simulink model "ADMIRE"  (R2021b)
settings: Solver=ode4  StartTime=0.0  StopTime=100  FixedStep=1e-2  RelTol=1e-3
undefined symbols (not defined in the file or in its folder): admireDB, Earth, WGS84
libraries: simulink_extras x112, simulink x27, aerolibutil x4, dspsigops x4, aerolibfltsims x3, sharedtransform x2, aerolibtransform2 x2, aerolibatmos2 x1, matrix_library x1, sharedutil x1, aerolibanimutils x1, vrlib x1
(part 6 of 15)

== system ADMIRE/Aircraft/Aerodynamics/PitchMomentCoefficient/MachRegion3/Cpmalfa ==
  in_bus : Inport
  Bus Selector : BusSelector  OutputSignals=AeroIn_Bus.angleOfAttack_deg,AeroIn_Bus.mach_nd,AeroIn_Bus.qacorr
  CPMEA_QA_M : Lookup_n-D  BreakpointsForDimension1=admireDB.aerodata_sym.CPMEA.breakpoints.M  BreakpointsForDimension2=admireDB.aerodata_sym.CPMEA.breakpoints.QA  BreakpointsForDimension3=[5, 7]  Table=admireDB.aerodata_sym.CPMEA.newTable  ExtrapMethod=Clip  InternalRulePriority=Speed  RndMeth=Simplest  InputSameDT=on
      settings: InputPortMap=u0,u1
  CPMMDEA_ALFA_DE_M : Lookup_n-D  NumberOfTableDimensions=3  BreakpointsForDimension1=admireDB.aerodata_sym.CPMMDEA.breakpoints.ALFA  BreakpointsForDimension2=admireDB.aerodata_sym.CPMMDEA.breakpoints.DE  BreakpointsForDimension3=admireDB.aerodata_sym.CPMMDEA.breakpoints.M  Table=admireDB.aerodata_sym.CPMMDEA.newTable  ExtrapMethod=Clip  InternalRulePriority=Speed  RndMeth=Simplest  InputSameDT=on
      settings: InputPortMap=u0,u1,u2
  Degrees to Radians : simulink_extras/Transformations/Degrees to Radians
  Product : Product
  Sum1 : Sum  Inputs=|++
  dE_cnst : Constant  Value=0.0
  Cpmalfa : Outport
  wires:
  Product/1 -> Sum1/2
  CPMMDEA_ALFA_DE_M/1 -> Sum1/1
  Sum1/1 -> Cpmalfa/1
  in_bus/1 -> Bus Selector/1  "in_bus"
  Bus Selector/1 -> CPMMDEA_ALFA_DE_M/1, Degrees to Radians/1  "<angleOfAttack_deg>"
  dE_cnst/1 -> CPMMDEA_ALFA_DE_M/2
  Bus Selector/3 -> CPMEA_QA_M/2  "<qacorr>"
  Bus Selector/2 -> CPMMDEA_ALFA_DE_M/3, CPMEA_QA_M/1  "<mach_nd>"
  CPMEA_QA_M/1 -> Product/2
  Degrees to Radians/1 -> Product/1

== system ADMIRE/Aircraft/Aerodynamics/PitchMomentCoefficient/MachRegion3/Cpmalfad ==
  in_bus : Inport
  Abs : Abs
  Bus Selector : BusSelector  OutputSignals=AeroIn_Bus.mach_nd,AeroIn_Bus.angleOfAttack_deg,AeroIn_Bus.alfad
  CPMADAM_ALFA_M : Lookup_n-D  BreakpointsForDimension1=admireDB.aerodata_sym.CPMADAM.breakpoints.M  BreakpointsForDimension2=admireDB.aerodata_sym.CPMADAM.breakpoints.ALFA  BreakpointsForDimension3=[5, 7]  Table=admireDB.aerodata_sym.CPMADAM.newTable  ExtrapMethod=Clip  InternalRulePriority=Speed  RndMeth=Simplest  InputSameDT=on
      settings: InputPortMap=u0,u1
  Product : Product
  Cpmalfad : Outport
  wires:
  in_bus/1 -> Bus Selector/1  "in_bus"
  Bus Selector/2 -> Abs/1  "<angleOfAttack_deg>"
  Bus Selector/1 -> CPMADAM_ALFA_M/1  "<mach_nd>"
  Abs/1 -> CPMADAM_ALFA_M/2
  CPMADAM_ALFA_M/1 -> Product/1
  Bus Selector/3 -> Product/2  "<alfad>"
  Product/1 -> Cpmalfad/1

== system ADMIRE/Aircraft/Aerodynamics/PitchMomentCoefficient/MachRegion3/Cpmbasic ==
  in_bus : Inport
  Bus Selector : BusSelector  OutputSignals=AeroIn_Bus.mach_nd,AeroIn_Bus.qacorr
  CPMEZERO_QA_M : Lookup_n-D  BreakpointsForDimension1=admireDB.aerodata_sym.CPMEZERO.breakpoints.M  BreakpointsForDimension2=admireDB.aerodata_sym.CPMEZERO.breakpoints.QA  BreakpointsForDimension3=[5, 7]  Table=admireDB.aerodata_sym.CPMEZERO.newTable  ExtrapMethod=Clip  InternalRulePriority=Speed  RndMeth=Simplest  InputSameDT=on
      settings: InputPortMap=u0,u1
  CPMZERO_M : Lookup_n-D  NumberOfTableDimensions=1  BreakpointsForDimension1=admireDB.aerodata_sym.CPMZERO.breakpoints.M  BreakpointsForDimension3=[5, 7]  Table=admireDB.aerodata_sym.CPMZERO.newTable  ExtrapMethod=Clip  InternalRulePriority=Speed  RndMeth=Simplest  InputSameDT=on
  Sum1 : Sum  Inputs=|++
  Cpmbasic : Outport
  wires:
  in_bus/1 -> Bus Selector/1  "in_bus"
  Sum1/1 -> Cpmbasic/1
  Bus Selector/1 -> CPMZERO_M/1, CPMEZERO_QA_M/1  "<mach_nd>"
  Bus Selector/2 -> CPMEZERO_QA_M/2  "<qacorr>"
  CPMZERO_M/1 -> Sum1/1
  CPMEZERO_QA_M/1 -> Sum1/2

== system ADMIRE/Aircraft/Aerodynamics/PitchMomentCoefficient/MachRegion3/Cpmbeta ==
  Constant : Constant  Value=0
  Cpmbeta : Outport
  wires:
  Constant/1 -> Cpmbeta/1

== system ADMIRE/Aircraft/Aerodynamics/PitchMomentCoefficient/MachRegion3/Cpmcai ==
  in_bus : Inport
  Bus Selector : BusSelector  OutputSignals=AeroIn_Bus.angleOfAttack_deg,AeroIn_Bus.cai,AeroIn_Bus.dN
  CPMCAIDN_ALFA_CAI_DN : Lookup_n-D  NumberOfTableDimensions=3  BreakpointsForDimension1=admireDB.aerodata_sym.CPMCAIDN.breakpoints.ALFA  BreakpointsForDimension2=admireDB.aerodata_sym.CPMCAIDN.breakpoints.CAI  BreakpointsForDimension3=admireDB.aerodata_sym.CPMCAIDN.breakpoints.DN  Table=admireDB.aerodata_sym.CPMCAIDN.newTable  ExtrapMethod=Clip  InternalRulePriority=Speed  RndMeth=Simplest  InputSameDT=on
      settings: InputPortMap=u0,u1,u2
  CPMCAI_CAI_ALFA : Lookup_n-D  BreakpointsForDimension1=admireDB.aerodata_sym.CPMCAI.breakpoints.ALFA  BreakpointsForDimension2=admireDB.aerodata_sym.CPMCAI.breakpoints.CAI  BreakpointsForDimension3=[5, 7]  Table=admireDB.aerodata_sym.CPMCAI.newTable  ExtrapMethod=Clip  InternalRulePriority=Speed  RndMeth=Simplest  InputSameDT=on
      settings: InputPortMap=u0,u1
  Sum : Sum  Inputs=|++
  Cpmcai : Outport
  wires:
  Bus Selector/3 -> CPMCAIDN_ALFA_CAI_DN/3  "<dN>"
  CPMCAI_CAI_ALFA/1 -> Sum/1
  Bus Selector/2 -> CPMCAI_CAI_ALFA/2, CPMCAIDN_ALFA_CAI_DN/2  "<cai>"
  Bus Selector/1 -> CPMCAI_CAI_ALFA/1, CPMCAIDN_ALFA_CAI_DN/1  "<angleOfAttack_deg>"
  in_bus/1 -> Bus Selector/1  "in_bus"
  Sum/1 -> Cpmcai/1
  CPMCAIDN_ALFA_CAI_DN/1 -> Sum/2

== system ADMIRE/Aircraft/Aerodynamics/PitchMomentCoefficient/MachRegion3/Cpmda ==
  Constant : Constant  Value=0
  Cpmda : Outport
  wires:
  Constant/1 -> Cpmda/1

== system ADMIRE/Aircraft/Aerodynamics/PitchMomentCoefficient/MachRegion3/Cpmdedn ==
  Constant : Constant  Value=0
  Cpmdedn : Outport
  wires:
  Constant/1 -> Cpmdedn/1

== system ADMIRE/Aircraft/Aerodynamics/PitchMomentCoefficient/MachRegion3/Cpmdei ==
  in_bus : Inport
  Bus Selector : BusSelector  OutputSignals=AeroIn_Bus.dEI,AeroIn_Bus.angleOfAttack_deg,eieff,AeroIn_Bus.mach_nd,AeroIn_Bus.qacorr
  CPMEDEI_QA_M : Lookup_n-D  BreakpointsForDimension1=admireDB.aerodata_sym.CPMEDEI.breakpoints.M  BreakpointsForDimension2=admireDB.aerodata_sym.CPMEDEI.breakpoints.QA  BreakpointsForDimension3=[5, 7]  Table=admireDB.aerodata_sym.CPMEDEI.newTable  ExtrapMethod=Clip  InternalRulePriority=Speed  RndMeth=Simplest  InputSameDT=on
      settings: InputPortMap=u0,u1
  Product : Product
  Subsystem : Subsystem
  Cpmdei : Outport
  wires:
  in_bus/1 -> Bus Selector/1  "in_bus"
  Bus Selector/5 -> CPMEDEI_QA_M/2  "<qacorr>"
  Bus Selector/1 -> Subsystem/1(dEI)  "<dEI>"
  Bus Selector/2 -> Subsystem/2(angleOfAttack_deg)  "<angleOfAttack_deg>"
  Bus Selector/3 -> Subsystem/3(eieff)  "<eieff>"
  Bus Selector/4 -> Subsystem/4(mach_nd), CPMEDEI_QA_M/1  "<mach_nd>"
  CPMEDEI_QA_M/1 -> Product/2
  Subsystem/1(Out1) -> Product/1
  Product/1 -> Cpmdei/1

== system ADMIRE/Aircraft/Aerodynamics/PitchMomentCoefficient/MachRegion3/Cpmdey ==
  in_bus : Inport
  Bus Selector : BusSelector  OutputSignals=AeroIn_Bus.dEY,AeroIn_Bus.angleOfAttack_deg,eoeff,AeroIn_Bus.mach_nd,AeroIn_Bus.qacorr
  CPMEDEY_QA_M : Lookup_n-D  BreakpointsForDimension1=admireDB.aerodata_sym.CPMEDEY.breakpoints.M  BreakpointsForDimension2=admireDB.aerodata_sym.CPMEDEY.breakpoints.QA  BreakpointsForDimension3=[5, 7]  Table=admireDB.aerodata_sym.CPMEDEY.newTable  ExtrapMethod=Clip  InternalRulePriority=Speed  RndMeth=Simplest  InputSameDT=on
      settings: InputPortMap=u0,u1
  Product : Product
  Subsystem : Subsystem
  Cpmdey : Outport
  wires:
  Product/1 -> Cpmdey/1
  Subsystem/1(Out1) -> Product/1
  CPMEDEY_QA_M/1 -> Product/2
  Bus Selector/4 -> Subsystem/4(mach_nd), CPMEDEY_QA_M/1  "<mach_nd>"
  Bus Selector/3 -> Subsystem/3(eoeff)  "<eoeff>"
  Bus Selector/2 -> Subsystem/2(angleOfAttack_deg)  "<angleOfAttack_deg>"
  Bus Selector/1 -> Subsystem/1(dEY)  "<dEY>"
  Bus Selector/5 -> CPMEDEY_QA_M/2  "<qacorr>"
  in_bus/1 -> Bus Selector/1  "in_bus"

== system ADMIRE/Aircraft/Aerodynamics/PitchMomentCoefficient/MachRegion3/Cpmdle ==
  in_bus : Inport
  Bus Selector : BusSelector  OutputSignals=AeroIn_Bus.angleOfAttack_deg,AeroIn_Bus.lef_deg,AeroIn_Bus.qacorr,AeroIn_Bus.mach_nd
  CPMMDLEA_ALFA_DLE_M : Lookup_n-D  NumberOfTableDimensions=3  BreakpointsForDimension1=admireDB.aerodata_sym.CPMMDLEA.breakpoints.ALFA  BreakpointsForDimension2=admireDB.aerodata_sym.CPMMDLEA.breakpoints.DLE  BreakpointsForDimension3=admireDB.aerodata_sym.CPMMDLEA.breakpoints.M  Table=admireDB.aerodata_sym.CPMMDLEA.newTable  ExtrapMethod=Clip  InternalRulePriority=Speed  RndMeth=Simplest  InputSameDT=on
      settings: InputPortMap=u0,u1,u2
  Degrees to Radians : simulink_extras/Transformations/Degrees to Radians
  Product : Product
  Subsystem1 : Subsystem
  Sum : Sum  Inputs=|++
  Cpmdle : Outport
  wires:
  in_bus/1 -> Bus Selector/1  "in_bus"
  Bus Selector/1 -> CPMMDLEA_ALFA_DLE_M/1  "<angleOfAttack_deg>"
  Bus Selector/2 -> CPMMDLEA_ALFA_DLE_M/2, Degrees to Radians/1  "<lef_deg>"
  Degrees to Radians/1 -> Product/2
  Product/1 -> Sum/2
  CPMMDLEA_ALFA_DLE_M/1 -> Sum/1
  Sum/1 -> Cpmdle/1
  Bus Selector/3 -> Subsystem1/1(<qacorr>)  "<qacorr>"
  Bus Selector/4 -> Subsystem1/2(<mach_nd>), CPMMDLEA_ALFA_DLE_M/3  "<mach_nd>"
  Subsystem1/1(Out1) -> Product/1

== system ADMIRE/Aircraft/Aerodynamics/PitchMomentCoefficient/MachRegion3/Cpmdn ==
  in_bus : Inport
  Bus Selector : BusSelector  OutputSignals=AeroIn_Bus.angleOfAttack_deg,AeroIn_Bus.dN,AeroIn_Bus.mach_nd,AeroIn_Bus.qacorr
  CPMEDN_QA_M : Lookup_n-D  BreakpointsForDimension1=admireDB.aerodata_sym.CPMEDN.breakpoints.M  BreakpointsForDimension2=admireDB.aerodata_sym.CPMEDN.breakpoints.QA  BreakpointsForDimension3=[5, 7]  Table=admireDB.aerodata_sym.CPMEDN.newTable  ExtrapMethod=Clip  InternalRulePriority=Speed  RndMeth=Simplest  InputSameDT=on
      settings: InputPortMap=u0,u1
  CPMMDNA_ALFA_DN_M : Lookup_n-D  NumberOfTableDimensions=3  BreakpointsForDimension1=admireDB.aerodata_sym.CPMMDNA.breakpoints.ALFA  BreakpointsForDimension2=admireDB.aerodata_sym.CPMMDNA.breakpoints.DN  BreakpointsForDimension3=admireDB.aerodata_sym.CPMMDNA.breakpoints.M  Table=admireDB.aerodata_sym.CPMMDNA.newTable  ExtrapMethod=Clip  InternalRulePriority=Speed  RndMeth=Simplest  InputSameDT=on
      settings: InputPortMap=u0,u1,u2
  Product : Product
  Cpmdn : Outport
  wires:
  Product/1 -> Cpmdn/1
  in_bus/1 -> Bus Selector/1  "in_bus"
  Bus Selector/1 -> CPMMDNA_ALFA_DN_M/1  "<angleOfAttack_deg>"
  Bus Selector/2 -> CPMMDNA_ALFA_DN_M/2  "<dN>"
  Bus Selector/4 -> CPMEDN_QA_M/2  "<qacorr>"
  Bus Selector/3 -> CPMMDNA_ALFA_DN_M/3, CPMEDN_QA_M/1  "<mach_nd>"
  CPMEDN_QA_M/1 -> Product/2
  CPMMDNA_ALFA_DN_M/1 -> Product/1

== system ADMIRE/Aircraft/Aerodynamics/PitchMomentCoefficient/MachRegion3/Cpmhigh ==
  Constant : Constant  Value=0
  Cpmhigh : Outport
  wires:
  Constant/1 -> Cpmhigh/1

== system ADMIRE/Aircraft/Aerodynamics/PitchMomentCoefficient/MachRegion3/Cpmlg ==
  in_bus : Inport
  Abs : Abs
  Bus Selector : BusSelector  OutputSignals=AeroIn_Bus.angleOfAttack_deg,AeroIn_Bus.angleOfSideslip_deg,AeroIn_Bus.lg_bool
  CPMLST_BETA_ALFA : Lookup_n-D  BreakpointsForDimension1=admireDB.aerodata_sym.CPMLST.breakpoints.ALFA  BreakpointsForDimension2=admireDB.aerodata_sym.CPMLST.breakpoints.BETA  BreakpointsForDimension3=[5, 7]  Table=admireDB.aerodata_sym.CPMLST.newTable  ExtrapMethod=Clip  InternalRulePriority=Speed  RndMeth=Simplest  InputSameDT=on
      settings: InputPortMap=u0,u1
  Product : Product
  Cpmlg : Outport
  wires:
  Product/1 -> Cpmlg/1
  in_bus/1 -> Bus Selector/1  "in_bus"
  Bus Selector/1 -> CPMLST_BETA_ALFA/1  "<angleOfAttack_deg>"
  Bus Selector/2 -> Abs/1  "<angleOfSideslip_deg>"
  CPMLST_BETA_ALFA/1 -> Product/1
  Bus Selector/3 -> Product/2  "<lg_bool>"
  Abs/1 -> CPMLST_BETA_ALFA/2

== system ADMIRE/Aircraft/Aerodynamics/PitchMomentCoefficient/MachRegion3/Cpmnz ==
  in_bus : Inport
  Bus Selector : BusSelector  OutputSignals=AeroIn_Bus.nz_g,AeroIn_Bus.mach_nd,AeroIn_Bus.qacorr
  CPMENZ_QA_M : Lookup_n-D  BreakpointsForDimension1=admireDB.aerodata_sym.CPMENZ.breakpoints.M  BreakpointsForDimension2=admireDB.aerodata_sym.CPMENZ.breakpoints.QA  BreakpointsForDimension3=[5, 7]  Table=admireDB.aerodata_sym.CPMENZ.newTable  ExtrapMethod=Clip  InternalRulePriority=Speed  RndMeth=Simplest  InputSameDT=on
      settings: InputPortMap=u0,u1
  Constant : Constant
  Product : Product
  Sum : Sum  Inputs=-+|
  Cpmnz : Outport
  wires:
  in_bus/1 -> Bus Selector/1  "in_bus"
  Sum/1 -> Product/1
  Product/1 -> Cpmnz/1
  Bus Selector/3 -> CPMENZ_QA_M/2  "<qacorr>"
  Bus Selector/2 -> CPMENZ_QA_M/1  "<mach_nd>"
  Bus Selector/1 -> Sum/2  "<nz_g>"
  Constant/1 -> Sum/1
  CPMENZ_QA_M/1 -> Product/2

== system ADMIRE/Aircraft/Aerodynamics/PitchMomentCoefficient/MachRegion3/Cpmq ==
  in_bus : Inport
  Bus Selector : BusSelector  OutputSignals=AeroIn_Bus.qc,AeroIn_Bus.mach_nd,AeroIn_Bus.qacorr,AeroIn_Bus.angleOfAttack_deg
  CPMEQ_QA_M : Lookup_n-D  BreakpointsForDimension1=admireDB.aerodata_sym.CPMEQ.breakpoints.M  BreakpointsForDimension2=admireDB.aerodata_sym.CPMEQ.breakpoints.QA  BreakpointsForDimension3=[5, 7]  Table=admireDB.aerodata_sym.CPMEQ.newTable  ExtrapMethod=Clip  InternalRulePriority=Speed  RndMeth=Simplest  InputSameDT=on
      settings: InputPortMap=u0,u1
  CPMQAM_ALFA_M : Lookup_n-D  BreakpointsForDimension1=admireDB.aerodata_sym.CPMQAM.breakpoints.M  BreakpointsForDimension2=admireDB.aerodata_sym.CPMQAM.breakpoints.ALFA  BreakpointsForDimension3=[5, 7]  Table=admireDB.aerodata_sym.CPMQAM.newTable  ExtrapMethod=Clip  InternalRulePriority=Speed  RndMeth=Simplest  InputSameDT=on
      settings: InputPortMap=u0,u1
  Product : Product  Inputs=3
  Cpmq : Outport
  wires:
  Bus Selector/1 -> Product/1  "<qc>"
  CPMEQ_QA_M/1 -> Product/2
  CPMQAM_ALFA_M/1 -> Product/3
  Product/1 -> Cpmq/1
  in_bus/1 -> Bus Selector/1  "in_bus"
  Bus Selector/4 -> CPMQAM_ALFA_M/2  "<angleOfAttack_deg>"
  Bus Selector/3 -> CPMEQ_QA_M/2  "<qacorr>"
  Bus Selector/2 -> CPMQAM_ALFA_M/1, CPMEQ_QA_M/1  "<mach_nd>"

== system ADMIRE/Aircraft/Aerodynamics/PitchMomentCoefficient/MachRegion3/Cpmqd ==
  in_bus : Inport
  Bus Selector : BusSelector  OutputSignals=AeroIn_Bus.qd,AeroIn_Bus.mach_nd,AeroIn_Bus.qacorr
  CPMEQD_QA_M : Lookup_n-D  BreakpointsForDimension1=admireDB.aerodata_sym.CPMEQD.breakpoints.M  BreakpointsForDimension2=admireDB.aerodata_sym.CPMEQD.breakpoints.QA  BreakpointsForDimension3=[5, 7]  Table=admireDB.aerodata_sym.CPMEQD.newTable  ExtrapMethod=Clip  InternalRulePriority=Speed  RndMeth=Simplest  InputSameDT=on
      settings: InputPortMap=u0,u1
  Product : Product
  Cpmqd : Outport
  wires:
  CPMEQD_QA_M/1 -> Product/2
  Bus Selector/1 -> Product/1  "<qd>"
  Bus Selector/2 -> CPMEQD_QA_M/1  "<mach_nd>"
  Bus Selector/3 -> CPMEQD_QA_M/2  "<qacorr>"
  Product/1 -> Cpmqd/1
  in_bus/1 -> Bus Selector/1  "in_bus"

== system ADMIRE/Aircraft/Aerodynamics/PitchMomentCoefficient/MachRegion3/eoeff ==
  AeroIn_Bus : Inport
  Abs : Abs
  Bus Selector : BusSelector  OutputSignals=mach_nd,angleOfAttack_deg
  CPMDEYOD_ALFA_M : Lookup_n-D  BreakpointsForDimension1=admireDB.aerodata_sym.CPMDEYOD.breakpoints.M  BreakpointsForDimension2=admireDB.aerodata_sym.CPMDEYOD.breakpoints.ALFA  BreakpointsForDimension3=[5, 7]  Table=admireDB.aerodata_sym.CPMDEYOD.newTable  ExtrapMethod=Clip  InternalRulePriority=Speed  RndMeth=Simplest  InputSameDT=on
      settings: InputPortMap=u0,u1
  Constant : Constant
  Sum : Sum  Inputs=-+|
  eoeff : Outport
  eieff : Outport  Port=2
  wires:
  AeroIn_Bus/1 -> Bus Selector/1
  Bus Selector/1 -> CPMDEYOD_ALFA_M/1  "<mach_nd>"
  Constant/1 -> Sum/2
  CPMDEYOD_ALFA_M/1 -> Sum/1, eoeff/1
  Sum/1 -> eieff/1
  Bus Selector/2 -> Abs/1  "<angleOfAttack_deg>"
  Abs/1 -> CPMDEYOD_ALFA_M/2

== system ADMIRE/Aircraft/Aerodynamics/RollMomentCoefficient/MachRegion1/Crmbasic ==
  in_bus : Inport
  Bus Selector : BusSelector  OutputSignals=AeroIn_Bus.angleOfAttack_deg
  Crmbasic_ : Subsystem
  Crmbasic : Outport
  wires:
  Crmbasic_/1(Crmbasic) -> Crmbasic/1
  Bus Selector/1 -> Crmbasic_/1(angleOfAttack_deg)  "<angleOfAttack_deg>"
  in_bus/1 -> Bus Selector/1  "in_bus"

== system ADMIRE/Aircraft/Aerodynamics/RollMomentCoefficient/MachRegion1/Crmbde ==
  in_bus : Inport
  Bus Selector : BusSelector  OutputSignals=AeroIn_Bus.angleOfAttack_deg,AeroIn_Bus.dN,AeroIn_Bus.dEI,AeroIn_Bus.angleOfSideslip_deg,AeroIn_Bus.dEY,eieff,eoeff
  Crmbde_ : Subsystem
  Crmbde : Outport
  wires:
  Bus Selector/7 -> Crmbde_/7(eoeff)  "<eoeff>"
  Bus Selector/6 -> Crmbde_/6(eieff)  "<eieff>"
  Bus Selector/5 -> Crmbde_/5(dEY)  "<dEY>"
  Bus Selector/4 -> Crmbde_/4(angleOfSideslip_deg)  "<angleOfSideslip_deg>"
  Bus Selector/3 -> Crmbde_/3(dEI)  "<dEI>"
  Bus Selector/2 -> Crmbde_/2(dN)  "<dN>"
  Bus Selector/1 -> Crmbde_/1(angleOfAttack_deg)  "<angleOfAttack_deg>"
  Crmbde_/1(Crmbde) -> Crmbde/1
  in_bus/1 -> Bus Selector/1  "in_bus"

== system ADMIRE/Aircraft/Aerodynamics/RollMomentCoefficient/MachRegion1/Crmbdle ==
  in_bus : Inport
  Bus Selector : BusSelector  OutputSignals=AeroIn_Bus.lef_deg,AeroIn_Bus.angleOfSideslip_deg,AeroIn_Bus.dEI,AeroIn_Bus.angleOfAttack_deg,AeroIn_Bus.dEY,eieff,eoeff
  Crmbdle_ : Subsystem
  Crmbdle : Outport
  wires:
  Bus Selector/7 -> Crmbdle_/7(eoeff)  "<eoeff>"
  Bus Selector/6 -> Crmbdle_/6(eieff)  "<eieff>"
  Bus Selector/5 -> Crmbdle_/5(dEY)  "<dEY>"
  Bus Selector/4 -> Crmbdle_/4(angleOfAttack_deg)  "<angleOfAttack_deg>"
  Bus Selector/3 -> Crmbdle_/3(dEI)  "<dEI>"
  Bus Selector/2 -> Crmbdle_/2(angleOfSideslip_deg)  "<angleOfSideslip_deg>"
  Bus Selector/1 -> Crmbdle_/1(dLE)  "<lef_deg>"
  Crmbdle_/1(Crmbdle) -> Crmbdle/1
  in_bus/1 -> Bus Selector/1  "in_bus"

== system ADMIRE/Aircraft/Aerodynamics/RollMomentCoefficient/MachRegion1/Crmbdn ==
  in_bus : Inport
  Bus Selector : BusSelector  OutputSignals=AeroIn_Bus.angleOfAttack_deg,AeroIn_Bus.dN,AeroIn_Bus.angleOfSideslip_deg
  Crmbdn_ : Subsystem
  Crmbdn : Outport
  wires:
  Bus Selector/1 -> Crmbdn_/1(angleOfAttack_deg)  "<angleOfAttack_deg>"
  Bus Selector/3 -> Crmbdn_/3(angleOfSideslip_deg)  "<angleOfSideslip_deg>"
  Bus Selector/2 -> Crmbdn_/2(dN)  "<dN>"
  in_bus/1 -> Bus Selector/1  "in_bus"
  Crmbdn_/1(Crmbdn) -> Crmbdn/1

== system ADMIRE/Aircraft/Aerodynamics/RollMomentCoefficient/MachRegion1/Crmbeta ==
  in_bus : Inport
  Bus Selector : BusSelector  OutputSignals=AeroIn_Bus.angleOfSideslip_deg,AeroIn_Bus.angleOfAttack_deg,AeroIn_Bus.qacorr,AeroIn_Bus.mach_nd
  Crmbeta_ : Subsystem
  Crmbeta : Outport
  wires:
  Bus Selector/4 -> Crmbeta_/4(mach_nd)  "<mach_nd>"
  Bus Selector/3 -> Crmbeta_/3(qacorr)  "<qacorr>"
  Bus Selector/2 -> Crmbeta_/2(angleOfAttack_deg)  "<angleOfAttack_deg>"
  Bus Selector/1 -> Crmbeta_/1(angleOfSideslip_deg)  "<angleOfSideslip_deg>"
  in_bus/1 -> Bus Selector/1  "in_bus"
  Crmbeta_/1(Crmbeta) -> Crmbeta/1

== system ADMIRE/Aircraft/Aerodynamics/RollMomentCoefficient/MachRegion1/Crmbetad ==
  in_bus : Inport
  Bus Selector : BusSelector  OutputSignals=AeroIn_Bus.angleOfAttack_deg,AeroIn_Bus.betad
  Crmbetad_ : Subsystem
  Crmbetad : Outport
  wires:
  Bus Selector/1 -> Crmbetad_/1(angleOfAttack_deg)  "<angleOfAttack_deg>"
  Bus Selector/2 -> Crmbetad_/2(betad)  "<betad>"
  in_bus/1 -> Bus Selector/1  "in_bus"
  Crmbetad_/1(Crmbetad) -> Crmbetad/1

== system ADMIRE/Aircraft/Aerodynamics/RollMomentCoefficient/MachRegion1/Crmblg ==
  in_bus : Inport
  Bus Selector : BusSelector  OutputSignals=AeroIn_Bus.lg_bool,AeroIn_Bus.angleOfAttack_deg,AeroIn_Bus.angleOfSideslip_deg
  Crmblg_ : Subsystem
  Crmblg : Outport
  wires:
  Bus Selector/3 -> Crmblg_/3(angleOfSideslip_deg)  "<angleOfSideslip_deg>"
  Bus Selector/2 -> Crmblg_/2(angleOfAttack_deg)  "<angleOfAttack_deg>"
  Bus Selector/1 -> Crmblg_/1(dLG)  "<lg_bool>"
  in_bus/1 -> Bus Selector/1  "in_bus"
  Crmblg_/1(Crmblg) -> Crmblg/1

== system ADMIRE/Aircraft/Aerodynamics/RollMomentCoefficient/MachRegion1/Crmdai ==
  in_bus : Inport
  Bus Selector : BusSelector  OutputSignals=AeroIn_Bus.dAI,AeroIn_Bus.angleOfAttack_deg,AeroIn_Bus.dEI,eieff,AeroIn_Bus.qacorr,AeroIn_Bus.mach_nd
  Crmdai_ : Subsystem
  Crmdai : Outport
  wires:
  Bus Selector/1 -> Crmdai_/1(dAI)  "<dAI>"
  Bus Selector/2 -> Crmdai_/2(angleOfAttack_deg)  "<angleOfAttack_deg>"
  Bus Selector/3 -> Crmdai_/3(dEI)  "<dEI>"
  Bus Selector/4 -> Crmdai_/4(eieff)  "<eieff>"
  Bus Selector/5 -> Crmdai_/5(qacorr)  "<qacorr>"
  Bus Selector/6 -> Crmdai_/6(mach_nd)  "<mach_nd>"
  in_bus/1 -> Bus Selector/1  "in_bus"
  Crmdai_/1(Crmdai) -> Crmdai/1

== system ADMIRE/Aircraft/Aerodynamics/RollMomentCoefficient/MachRegion1/Crmdaib ==
  in_bus : Inport
  Bus Selector : BusSelector  OutputSignals=AeroIn_Bus.angleOfAttack_deg,AeroIn_Bus.dAI,AeroIn_Bus.angleOfSideslip_deg,eieff
  Crmdaib_ : Subsystem
  Crmdaib : Outport
  wires:
  Bus Selector/1 -> Crmdaib_/1(angleOfAttack_deg)  "<angleOfAttack_deg>"
  Bus Selector/2 -> Crmdaib_/2(dAI)  "<dAI>"
  Bus Selector/3 -> Crmdaib_/3(angleOfSideslip_deg)  "<angleOfSideslip_deg>"
  Bus Selector/4 -> Crmdaib_/4(eieff)  "<eieff>"
  Crmdaib_/1(Crmdaib) -> Crmdaib/1
  in_bus/1 -> Bus Selector/1  "in_bus"

== system ADMIRE/Aircraft/Aerodynamics/RollMomentCoefficient/MachRegion1/Crmday ==
  in_bus : Inport
  Bus Selector : BusSelector  OutputSignals=AeroIn_Bus.dAY,AeroIn_Bus.angleOfAttack_deg,AeroIn_Bus.dEY,eoeff,AeroIn_Bus.qacorr,AeroIn_Bus.mach_nd
  Crmday_ : Subsystem
  Crmday : Outport
  wires:
  Crmday_/1(Crmdai) -> Crmday/1
  in_bus/1 -> Bus Selector/1  "in_bus"
  Bus Selector/6 -> Crmday_/6(mach_nd)  "<mach_nd>"
  Bus Selector/5 -> Crmday_/5(qacorr)  "<qacorr>"
  Bus Selector/4 -> Crmday_/4(eoeff)  "<eoeff>"
  Bus Selector/3 -> Crmday_/3(dEY)  "<dEY>"
  Bus Selector/2 -> Crmday_/2(angleOfAttack_deg)  "<angleOfAttack_deg>"
  Bus Selector/1 -> Crmday_/1(dAY)  "<dAY>"

== system ADMIRE/Aircraft/Aerodynamics/RollMomentCoefficient/MachRegion1/Crmdayb ==
  in_bus : Inport
  Bus Selector : BusSelector  OutputSignals=AeroIn_Bus.angleOfAttack_deg,AeroIn_Bus.dAY,AeroIn_Bus.angleOfSideslip_deg,eoeff
  Crmdaib_ : Subsystem
  Crmdayb : Outport
  wires:
  in_bus/1 -> Bus Selector/1  "in_bus"
  Crmdaib_/1(Crmdaib) -> Crmdayb/1
  Bus Selector/4 -> Crmdaib_/4(eoeff)  "<eoeff>"
  Bus Selector/3 -> Crmdaib_/3(angleOfSideslip_deg)  "<angleOfSideslip_deg>"
  Bus Selector/2 -> Crmdaib_/2(dAY)  "<dAY>"
  Bus Selector/1 -> Crmdaib_/1(angleOfAttack_deg)  "<angleOfAttack_deg>"

== system ADMIRE/Aircraft/Aerodynamics/RollMomentCoefficient/MachRegion1/Crmdna ==
  in_bus : Inport
  Bus Selector : BusSelector  OutputSignals=AeroIn_Bus.dNE,AeroIn_Bus.angleOfAttack_deg,AeroIn_Bus.dNA
  Crmdna_ : Subsystem
  Crmdna : Outport
  wires:
  Bus Selector/3 -> Crmdna_/3(dNA)  "<dNA>"
  Bus Selector/2 -> Crmdna_/2(angleOfAttack_deg)  "<angleOfAttack_deg>"
  Bus Selector/1 -> Crmdna_/1(dNE)  "<dNE>"
  Crmdna_/1(Crmdna) -> Crmdna/1
  in_bus/1 -> Bus Selector/1  "in_bus"

== system ADMIRE/Aircraft/Aerodynamics/RollMomentCoefficient/MachRegion1/Crmdr ==
  in_bus : Inport
  Bus Selector : BusSelector  OutputSignals=AeroIn_Bus.angleOfAttack_deg,AeroIn_Bus.rud_deg,AeroIn_Bus.angleOfSideslip_deg,AeroIn_Bus.qacorr,AeroIn_Bus.mach_nd
  Crmdr_ : Subsystem
  Crmdr : Outport
  wires:
  Bus Selector/5 -> Crmdr_/5(mach_nd)  "<mach_nd>"
  Bus Selector/4 -> Crmdr_/4(qacorr)  "<qacorr>"
  Bus Selector/3 -> Crmdr_/3(angleOfSideslip_deg)  "<angleOfSideslip_deg>"
  Bus Selector/2 -> Crmdr_/2(dR)  "<rud_deg>"
  Bus Selector/1 -> Crmdr_/1(angleOfAttack_deg)  "<angleOfAttack_deg>"
  Crmdr_/1(Crmdr) -> Crmdr/1
  in_bus/1 -> Bus Selector/1  "in_bus"

== system ADMIRE/Aircraft/Aerodynamics/RollMomentCoefficient/MachRegion1/Crmp ==
  in_bus : Inport
  Bus Selector : BusSelector  OutputSignals=AeroIn_Bus.dN,AeroIn_Bus.angleOfAttack_deg,AeroIn_Bus.qacorr,AeroIn_Bus.mach_nd,AeroIn_Bus.pc
  Crmp_ : Subsystem
  Crmp : Outport
  wires:
  Bus Selector/1 -> Crmp_/1(dN)  "<dN>"
  Bus Selector/2 -> Crmp_/2(angleOfAttack_deg)  "<angleOfAttack_deg>"
  Bus Selector/3 -> Crmp_/3(qacorr)  "<qacorr>"
  Bus Selector/4 -> Crmp_/4(mach_nd)  "<mach_nd>"
  Bus Selector/5 -> Crmp_/5(pc)  "<pc>"
  Crmp_/1(Crmp) -> Crmp/1
  in_bus/1 -> Bus Selector/1  "in_bus"

== system ADMIRE/Aircraft/Aerodynamics/RollMomentCoefficient/MachRegion1/Crmpbeta ==
  in_bus : Inport
  Bus Selector : BusSelector  OutputSignals=AeroIn_Bus.angleOfSideslip_deg,AeroIn_Bus.angleOfAttack_deg,AeroIn_Bus.pc
  Crmpbeta_ : Subsystem
  Crmpbeta : Outport
  wires:
  Bus Selector/1 -> Crmpbeta_/1(angleOfSideslip_deg)  "<angleOfSideslip_deg>"
  Bus Selector/2 -> Crmpbeta_/2(angleOfAttack_deg)  "<angleOfAttack_deg>"
  Bus Selector/3 -> Crmpbeta_/3(pc)  "<pc>"
  in_bus/1 -> Bus Selector/1  "in_bus"
  Crmpbeta_/1(Crmpbeta) -> Crmpbeta/1

== system ADMIRE/Aircraft/Aerodynamics/RollMomentCoefficient/MachRegion1/Crmr ==
  in_bus : Inport
  Bus Selector : BusSelector  OutputSignals=AeroIn_Bus.dN,AeroIn_Bus.angleOfAttack_deg,AeroIn_Bus.rc
  Crmr_ : Subsystem
  Crmr : Outport
  wires:
  Bus Selector/1 -> Crmr_/1(dN)  "<dN>"
  Bus Selector/2 -> Crmr_/2(angleOfAttack_deg)  "<angleOfAttack_deg>"
  Bus Selector/3 -> Crmr_/3(rc)  "<rc>"
  Crmr_/1(Crmr) -> Crmr/1
  in_bus/1 -> Bus Selector/1  "in_bus"

== system ADMIRE/Aircraft/Aerodynamics/RollMomentCoefficient/MachRegion1/Crmrbeta ==
  in_bus : Inport
  Bus Selector : BusSelector  OutputSignals=AeroIn_Bus.angleOfSideslip_deg,AeroIn_Bus.angleOfAttack_deg,AeroIn_Bus.rc
  Crmrbeta_ : Subsystem
  Crmrbeta : Outport
  wires:
  in_bus/1 -> Bus Selector/1  "in_bus"
  Crmrbeta_/1(Crmrbeta) -> Crmrbeta/1
  Bus Selector/3 -> Crmrbeta_/3(rc)  "<rc>"
  Bus Selector/2 -> Crmrbeta_/2(angleOfAttack_deg)  "<angleOfAttack_deg>"
  Bus Selector/1 -> Crmrbeta_/1(angleOfSideslip_deg)  "<angleOfSideslip_deg>"

== system ADMIRE/Aircraft/Aerodynamics/RollMomentCoefficient/MachRegion1/Crmrde ==
  in_bus : Inport
  Bus Selector : BusSelector  OutputSignals=AeroIn_Bus.mach_nd,AeroIn_Bus.angleOfAttack_deg,AeroIn_Bus.rc,AeroIn_Bus.dEI,eieff,AeroIn_Bus.dEY,eoeff
  Crmrde_ : Subsystem
  Crmrbeta : Outport
  wires:
  Bus Selector/1 -> Crmrde_/1(mach_nd)  "<mach_nd>"
  Bus Selector/2 -> Crmrde_/2(angleOfAttack_deg)  "<angleOfAttack_deg>"
  Bus Selector/3 -> Crmrde_/3(rc)  "<rc>"
  Bus Selector/4 -> Crmrde_/4(dEI)  "<dEI>"
  Bus Selector/5 -> Crmrde_/5(eieff)  "<eieff>"
  Bus Selector/6 -> Crmrde_/6(dey)  "<dEY>"
  Bus Selector/7 -> Crmrde_/7(eoeff)  "<eoeff>"
  Crmrde_/1(Crmrbeta) -> Crmrbeta/1
  in_bus/1 -> Bus Selector/1  "in_bus"

== system ADMIRE/Aircraft/Aerodynamics/RollMomentCoefficient/MachRegion1/eoeff1 ==
  AeroIn_Bus : Inport
  Bus Selector : BusSelector  OutputSignals=mach_nd
  CRMDAYOD_M : Lookup_n-D  NumberOfTableDimensions=1  BreakpointsForDimension1=admireDB.aerodata_asym_ext.CRMDAYOD.breakpoints.M  BreakpointsForDimension3=[5, 7]  Table=admireDB.aerodata_asym_ext.CRMDAYOD.newTable  ExtrapMethod=Clip  InternalRulePriority=Speed  RndMeth=Simplest  InputSameDT=on
  Constant : Constant
  Sum : Sum  Inputs=-+|
  eoeff : Outport
  eieff : Outport  Port=2
  wires:
  Sum/1 -> eieff/1
  CRMDAYOD_M/1 -> eoeff/1, Sum/1
  Constant/1 -> Sum/2
  Bus Selector/1 -> CRMDAYOD_M/1  "<mach_nd>"
  AeroIn_Bus/1 -> Bus Selector/1

== system ADMIRE/Aircraft/Aerodynamics/RollMomentCoefficient/MachRegion2/Crmbasic ==
  in_bus : Inport
  Bus Selector : BusSelector  OutputSignals=AeroIn_Bus.angleOfAttack_deg,AeroIn_Bus.tflow
  Crmbasic_ : Subsystem
  Crmbasic : Outport
  wires:
  Bus Selector/2 -> Crmbasic_/2(tflow)  "<tflow>"
  Crmbasic_/1(Crmbasic) -> Crmbasic/1
  Bus Selector/1 -> Crmbasic_/1(angleOfAttack_deg)  "<angleOfAttack_deg>"
  in_bus/1 -> Bus Selector/1  "in_bus"

== system ADMIRE/Aircraft/Aerodynamics/RollMomentCoefficient/MachRegion2/Crmbde ==
  in_bus : Inport
  Bus Selector : BusSelector  OutputSignals=AeroIn_Bus.angleOfAttack_deg,AeroIn_Bus.dN,AeroIn_Bus.dEI,AeroIn_Bus.angleOfSideslip_deg,AeroIn_Bus.dEY,eieff,eoeff
  Crmbde_ : Subsystem
  Crmbde : Outport
  wires:
  Bus Selector/1 -> Crmbde_/1(angleOfAttack_deg)  "<angleOfAttack_deg>"
  Bus Selector/2 -> Crmbde_/2(dN)  "<dN>"
  Bus Selector/3 -> Crmbde_/3(dEI)  "<dEI>"
  Bus Selector/4 -> Crmbde_/4(angleOfSideslip_deg)  "<angleOfSideslip_deg>"
  Bus Selector/5 -> Crmbde_/5(dEY)  "<dEY>"
  Bus Selector/6 -> Crmbde_/6(eieff)  "<eieff>"
  Bus Selector/7 -> Crmbde_/7(eoeff)  "<eoeff>"
  Crmbde_/1(Crmbde) -> Crmbde/1
  in_bus/1 -> Bus Selector/1  "in_bus"

== system ADMIRE/Aircraft/Aerodynamics/RollMomentCoefficient/MachRegion2/Crmbdle ==
  in_bus : Inport
  Bus Selector : BusSelector  OutputSignals=AeroIn_Bus.angleOfAttack_deg,AeroIn_Bus.dEI,AeroIn_Bus.angleOfSideslip_deg,AeroIn_Bus.lef_deg,AeroIn_Bus.dEY,AeroIn_Bus.tflow,AeroIn_Bus.tfhigh
  Crmbdle_ : Subsystem
  Crmbdle : Outport
  wires:
  Bus Selector/7 -> Crmbdle_/7(tfhigh)  "<tfhigh>"
  Bus Selector/6 -> Crmbdle_/6(tflow)  "<tflow>"
  Bus Selector/5 -> Crmbdle_/5(dEY)  "<dEY>"
  Bus Selector/4 -> Crmbdle_/4(dLE)  "<lef_deg>"
  Bus Selector/3 -> Crmbdle_/3(angleOfSideslip_deg)  "<angleOfSideslip_deg>"
  Bus Selector/2 -> Crmbdle_/2(dEI)  "<dEI>"
  Bus Selector/1 -> Crmbdle_/1(angleOfAttack_deg)  "<angleOfAttack_deg>"
  Crmbdle_/1(Crmbdle) -> Crmbdle/1
  in_bus/1 -> Bus Selector/1  "in_bus"

== system ADMIRE/Aircraft/Aerodynamics/RollMomentCoefficient/MachRegion2/Crmbdn ==
  in_bus : Inport
  Bus Selector : BusSelector  OutputSignals=AeroIn_Bus.angleOfSideslip_deg,AeroIn_Bus.dN,AeroIn_Bus.angleOfAttack_deg,AeroIn_Bus.tflow,AeroIn_Bus.tfhigh
  Crmbdn_ : Subsystem
  Crmbdn : Outport
  wires:
  Bus Selector/1 -> Crmbdn_/1(angleOfSideslip_deg)  "<angleOfSideslip_deg>"
  Bus Selector/2 -> Crmbdn_/2(dN)  "<dN>"
  Bus Selector/3 -> Crmbdn_/3(angleOfAttack_deg)  "<angleOfAttack_deg>"
  Bus Selector/4 -> Crmbdn_/4(tflow)  "<tflow>"
  Bus Selector/5 -> Crmbdn_/5(tfhigh)  "<tfhigh>"
  in_bus/1 -> Bus Selector/1  "in_bus"
  Crmbdn_/1(Crmbdn) -> Crmbdn/1

== system ADMIRE/Aircraft/Aerodynamics/RollMomentCoefficient/MachRegion2/Crmbeta ==
  in_bus : Inport
  Bus Selector : BusSelector  OutputSignals=AeroIn_Bus.angleOfSideslip_deg,AeroIn_Bus.angleOfAttack_deg,AeroIn_Bus.tflow,AeroIn_Bus.tfhigh,AeroIn_Bus.qacorr,AeroIn_Bus.mach_nd
  Crmbeta_ : Subsystem
  Crmbeta : Outport
  wires:
  Bus Selector/1 -> Crmbeta_/1(angleOfSideslip_deg)  "<angleOfSideslip_deg>"
  Bus Selector/2 -> Crmbeta_/2(angleOfAttack_deg)  "<angleOfAttack_deg>"
  Bus Selector/3 -> Crmbeta_/3(tflow)  "<tflow>"
  Bus Selector/4 -> Crmbeta_/4(thigh)  "<tfhigh>"
  Bus Selector/5 -> Crmbeta_/5(qacorr)  "<qacorr>"
  Bus Selector/6 -> Crmbeta_/6(mach_nd)  "<mach_nd>"
  in_bus/1 -> Bus Selector/1  "in_bus"
  Crmbeta_/1(Crmbeta) -> Crmbeta/1

== system ADMIRE/Aircraft/Aerodynamics/RollMomentCoefficient/MachRegion2/Crmbetad ==
  in_bus : Inport
  Bus Selector : BusSelector  OutputSignals=AeroIn_Bus.angleOfAttack_deg,AeroIn_Bus.betad,AeroIn_Bus.tflow,AeroIn_Bus.tfhigh
  Crmbetad_ : Subsystem
  Crmbetad : Outport
  wires:
  Bus Selector/1 -> Crmbetad_/1(angleOfAttack_deg)  "<angleOfAttack_deg>"
  Bus Selector/2 -> Crmbetad_/2(betad)  "<betad>"
  Bus Selector/3 -> Crmbetad_/3(tflow)  "<tflow>"
  Bus Selector/4 -> Crmbetad_/4(tfhigh)  "<tfhigh>"
  in_bus/1 -> Bus Selector/1  "in_bus"
  Crmbetad_/1(Crmbetad) -> Crmbetad/1

== system ADMIRE/Aircraft/Aerodynamics/RollMomentCoefficient/MachRegion2/Crmblg ==
  in_bus : Inport
  Bus Selector : BusSelector  OutputSignals=AeroIn_Bus.lg_bool,AeroIn_Bus.angleOfAttack_deg,AeroIn_Bus.angleOfSideslip_deg
  Crmblg_ : Subsystem
  Crmblg : Outport
  wires:
  Bus Selector/3 -> Crmblg_/3(angleOfSideslip_deg)  "<angleOfSideslip_deg>"
  Bus Selector/2 -> Crmblg_/2(angleOfAttack_deg)  "<angleOfAttack_deg>"
  Bus Selector/1 -> Crmblg_/1(dLG)  "<lg_bool>"
  in_bus/1 -> Bus Selector/1  "in_bus"
  Crmblg_/1(Crmblg) -> Crmblg/1

== system ADMIRE/Aircraft/Aerodynamics/RollMomentCoefficient/MachRegion2/Crmdai ==
  in_bus : Inport
  Bus Selector : BusSelector  OutputSignals=AeroIn_Bus.dAI,AeroIn_Bus.angleOfAttack_deg,AeroIn_Bus.dEI,eieff,AeroIn_Bus.qacorr,AeroIn_Bus.mach_nd,AeroIn_Bus.tflow,AeroIn_Bus.tfhigh
  Crmdai_ : Subsystem
  Crmdai : Outport
  wires:
  Bus Selector/8 -> Crmdai_/8(tfhigh)  "<tfhigh>"
  Bus Selector/7 -> Crmdai_/7(tflow)  "<tflow>"
  Bus Selector/6 -> Crmdai_/6(mach_nd)  "<mach_nd>"
  Bus Selector/5 -> Crmdai_/5(qacorr)  "<qacorr>"
  Bus Selector/4 -> Crmdai_/4(eieff)  "<eieff>"
  Bus Selector/3 -> Crmdai_/3(dEI)  "<dEI>"
  Bus Selector/2 -> Crmdai_/2(angleOfAttack_deg)  "<angleOfAttack_deg>"
  Bus Selector/1 -> Crmdai_/1(dAI)  "<dAI>"
  in_bus/1 -> Bus Selector/1  "in_bus"
  Crmdai_/1(Crmdai) -> Crmdai/1

== system ADMIRE/Aircraft/Aerodynamics/RollMomentCoefficient/MachRegion2/Crmdaib ==
  in_bus : Inport
  Bus Selector : BusSelector  OutputSignals=AeroIn_Bus.angleOfAttack_deg,AeroIn_Bus.dAI,AeroIn_Bus.angleOfSideslip_deg,eieff,AeroIn_Bus.tflow
  Crmdaib_ : Subsystem
  Crmdaib : Outport
  wires:
  Bus Selector/1 -> Crmdaib_/1(angleOfAttack_deg)  "<angleOfAttack_deg>"
  Bus Selector/2 -> Crmdaib_/2(dAI)  "<dAI>"
  Bus Selector/3 -> Crmdaib_/3(angleOfSideslip_deg)  "<angleOfSideslip_deg>"
  Bus Selector/4 -> Crmdaib_/4(eieff)  "<eieff>"
  Bus Selector/5 -> Crmdaib_/5(tflow)  "<tflow>"
  Crmdaib_/1(Crmdaib) -> Crmdaib/1
  in_bus/1 -> Bus Selector/1  "in_bus"

== system ADMIRE/Aircraft/Aerodynamics/RollMomentCoefficient/MachRegion2/Crmday ==
  in_bus : Inport
  Bus Selector : BusSelector  OutputSignals=AeroIn_Bus.dAY,AeroIn_Bus.angleOfAttack_deg,AeroIn_Bus.dEY,eoeff,AeroIn_Bus.qacorr,AeroIn_Bus.mach_nd,AeroIn_Bus.tflow,AeroIn_Bus.tfhigh
  Crmday_ : Subsystem
  Crmday : Outport
  wires:
  Bus Selector/8 -> Crmday_/8(tfhigh)  "<tfhigh>"
  Bus Selector/7 -> Crmday_/7(tflow)  "<tflow>"
  Bus Selector/6 -> Crmday_/6(mach_nd)  "<mach_nd>"
  Bus Selector/5 -> Crmday_/5(qacorr)  "<qacorr>"
  Bus Selector/4 -> Crmday_/4(eoeff)  "<eoeff>"
  Bus Selector/3 -> Crmday_/3(dEY)  "<dEY>"
  Bus Selector/2 -> Crmday_/2(angleOfAttack_deg)  "<angleOfAttack_deg>"
  Bus Selector/1 -> Crmday_/1(dAY)  "<dAY>"
  Crmday_/1(Crmdai) -> Crmday/1
  in_bus/1 -> Bus Selector/1  "in_bus"

== system ADMIRE/Aircraft/Aerodynamics/RollMomentCoefficient/MachRegion2/Crmdayb ==
  in_bus : Inport
  Bus Selector : BusSelector  OutputSignals=AeroIn_Bus.angleOfAttack_deg,AeroIn_Bus.dAY,AeroIn_Bus.angleOfSideslip_deg,eoeff,AeroIn_Bus.tflow
  Crmdayb_ : Subsystem
  Crmdayb : Outport
  wires:
  Bus Selector/5 -> Crmdayb_/5(tflow)  "<tflow>"
  Bus Selector/4 -> Crmdayb_/4(eoeff)  "<eoeff>"
  Bus Selector/3 -> Crmdayb_/3(angleOfSideslip_deg)  "<angleOfSideslip_deg>"
  Bus Selector/2 -> Crmdayb_/2(dAY)  "<dAY>"
  Bus Selector/1 -> Crmdayb_/1(angleOfAttack_deg)  "<angleOfAttack_deg>"
  in_bus/1 -> Bus Selector/1  "in_bus"
  Crmdayb_/1(Crmdayb) -> Crmdayb/1

== system ADMIRE/Aircraft/Aerodynamics/RollMomentCoefficient/MachRegion2/Crmdna ==
  in_bus : Inport
  Bus Selector : BusSelector  OutputSignals=AeroIn_Bus.dNE,AeroIn_Bus.angleOfAttack_deg,AeroIn_Bus.tflow,AeroIn_Bus.tfhigh,AeroIn_Bus.dNA
  Crmdna_ : Subsystem
  Crmdna : Outport
  wires:
  Bus Selector/1 -> Crmdna_/1(dNE)  "<dNE>"
  Bus Selector/2 -> Crmdna_/2(angleOfAttack_deg)  "<angleOfAttack_deg>"
  Bus Selector/3 -> Crmdna_/3(tflow)  "<tflow>"
  Bus Selector/4 -> Crmdna_/4(tfhigh)  "<tfhigh>"
  Bus Selector/5 -> Crmdna_/5(dNA)  "<dNA>"
  Crmdna_/1(Crmdna) -> Crmdna/1
  in_bus/1 -> Bus Selector/1  "in_bus"

== system ADMIRE/Aircraft/Aerodynamics/RollMomentCoefficient/MachRegion2/Crmdr ==
  in_bus : Inport
  Bus Selector : BusSelector  OutputSignals=AeroIn_Bus.angleOfAttack_deg,AeroIn_Bus.rud_deg,AeroIn_Bus.tfhigh,AeroIn_Bus.angleOfSideslip_deg,AeroIn_Bus.tflow,AeroIn_Bus.qacorr,AeroIn_Bus.mach_nd
  Crmdr_ : Subsystem
  Crmdr : Outport
  wires:
  Bus Selector/1 -> Crmdr_/1(angleOfAttack_deg)  "<angleOfAttack_deg>"
  Bus Selector/2 -> Crmdr_/2(dR)  "<rud_deg>"
  Bus Selector/7 -> Crmdr_/7(mach_nd)  "<mach_nd>"
  Bus Selector/3 -> Crmdr_/3(tfhigh)  "<tfhigh>"
  Bus Selector/6 -> Crmdr_/6(qacorr)  "<qacorr>"
  Bus Selector/4 -> Crmdr_/4(angleOfSideslip_deg)  "<angleOfSideslip_deg>"
  Bus Selector/5 -> Crmdr_/5(tflow)  "<tflow>"
  Crmdr_/1(Crmdr) -> Crmdr/1
  in_bus/1 -> Bus Selector/1  "in_bus"

== system ADMIRE/Aircraft/Aerodynamics/RollMomentCoefficient/MachRegion2/Crmp ==
  in_bus : Inport
  Bus Selector : BusSelector  OutputSignals=AeroIn_Bus.dN,AeroIn_Bus.angleOfAttack_deg,AeroIn_Bus.qacorr,AeroIn_Bus.mach_nd,AeroIn_Bus.pc,AeroIn_Bus.tflow,AeroIn_Bus.tfhigh
  Crmp_ : Subsystem
  Crmp : Outport
  wires:
  Bus Selector/7 -> Crmp_/7(tfhigh)  "<tfhigh>"
  Bus Selector/1 -> Crmp_/1(dN)  "<dN>"
  Bus Selector/6 -> Crmp_/6(tflow)  "<tflow>"
  Bus Selector/2 -> Crmp_/2(angleOfAttack_deg)  "<angleOfAttack_deg>"
  Bus Selector/5 -> Crmp_/5(pc)  "<pc>"
  Bus Selector/3 -> Crmp_/3(qacorr)  "<qacorr>"
  Bus Selector/4 -> Crmp_/4(mach_nd)  "<mach_nd>"
  Crmp_/1(Crmp) -> Crmp/1
  in_bus/1 -> Bus Selector/1  "in_bus"

== system ADMIRE/Aircraft/Aerodynamics/RollMomentCoefficient/MachRegion2/Crmpbeta ==
  in_bus : Inport
  Bus Selector : BusSelector  OutputSignals=AeroIn_Bus.angleOfSideslip_deg,AeroIn_Bus.pc,AeroIn_Bus.angleOfAttack_deg,AeroIn_Bus.tflow
  Crmpbeta_ : Subsystem
  Crmpbeta : Outport
  wires:
  Bus Selector/4 -> Crmpbeta_/4(tflow)  "<tflow>"
  Bus Selector/3 -> Crmpbeta_/3(angleOfAttack_deg)  "<angleOfAttack_deg>"
  Bus Selector/1 -> Crmpbeta_/1(angleOfSideslip_deg)  "<angleOfSideslip_deg>"
  Bus Selector/2 -> Crmpbeta_/2(pc)  "<pc>"
  in_bus/1 -> Bus Selector/1  "in_bus"
  Crmpbeta_/1(Crmpbeta) -> Crmpbeta/1

== system ADMIRE/Aircraft/Aerodynamics/RollMomentCoefficient/MachRegion2/Crmr ==
  in_bus : Inport
  Bus Selector : BusSelector  OutputSignals=AeroIn_Bus.dN,AeroIn_Bus.angleOfAttack_deg,AeroIn_Bus.rc,AeroIn_Bus.tflow,AeroIn_Bus.tfhigh
  Crmr_ : Subsystem
  Crmr : Outport
  wires:
  Bus Selector/5 -> Crmr_/5(tfhigh)  "<tfhigh>"
  Bus Selector/4 -> Crmr_/4(tflow)  "<tflow>"
  Bus Selector/3 -> Crmr_/3(rc)  "<rc>"
  Bus Selector/2 -> Crmr_/2(angleOfAttack_deg)  "<angleOfAttack_deg>"
  Bus Selector/1 -> Crmr_/1(dN)  "<dN>"
  Crmr_/1(Crmr) -> Crmr/1
  in_bus/1 -> Bus Selector/1  "in_bus"

== system ADMIRE/Aircraft/Aerodynamics/RollMomentCoefficient/MachRegion2/Crmrbeta ==
  in_bus : Inport
  Bus Selector : BusSelector  OutputSignals=AeroIn_Bus.angleOfSideslip_deg,AeroIn_Bus.angleOfAttack_deg,AeroIn_Bus.rc,AeroIn_Bus.tflow
  Crmrbeta_ : Subsystem
  Crmrbeta : Outport
  wires:
  Bus Selector/1 -> Crmrbeta_/1(angleOfSideslip_deg)  "<angleOfSideslip_deg>"
  Bus Selector/2 -> Crmrbeta_/2(angleOfAttack_deg)  "<angleOfAttack_deg>"
  Bus Selector/3 -> Crmrbeta_/3(rc)  "<rc>"
  Bus Selector/4 -> Crmrbeta_/4(tflow)  "<tflow>"
  in_bus/1 -> Bus Selector/1  "in_bus"
  Crmrbeta_/1(Crmrbeta) -> Crmrbeta/1

== system ADMIRE/Aircraft/Aerodynamics/RollMomentCoefficient/MachRegion2/Crmrde ==
  in_bus : Inport
  Bus Selector : BusSelector  OutputSignals=AeroIn_Bus.mach_nd,AeroIn_Bus.angleOfAttack_deg,AeroIn_Bus.rc,AeroIn_Bus.dEI,eieff,AeroIn_Bus.dEY,eoeff
  Crmrde_ : Subsystem
  Crmrde : Outport
  wires:
  Bus Selector/7 -> Crmrde_/7(eoeff)  "<eoeff>"
  Bus Selector/1 -> Crmrde_/1(mach_nd)  "<mach_nd>"
  Bus Selector/6 -> Crmrde_/6(dey)  "<dEY>"
  Bus Selector/2 -> Crmrde_/2(angleOfAttack_deg)  "<angleOfAttack_deg>"
  Bus Selector/5 -> Crmrde_/5(eieff)  "<eieff>"
  Bus Selector/3 -> Crmrde_/3(rc)  "<rc>"
  Bus Selector/4 -> Crmrde_/4(dEI)  "<dEI>"
  Crmrde_/1(Crmrde) -> Crmrde/1
  in_bus/1 -> Bus Selector/1  "in_bus"

== system ADMIRE/Aircraft/Aerodynamics/RollMomentCoefficient/MachRegion2/eoeff1 ==
  AeroIn_Bus : Inport
  Bus Selector : BusSelector  OutputSignals=mach_nd
  CRMDAYOD_M : Lookup_n-D  NumberOfTableDimensions=1  BreakpointsForDimension1=admireDB.aerodata_asym_ext.CRMDAYOD.breakpoints.M  BreakpointsForDimension3=[5, 7]  Table=admireDB.aerodata_asym_ext.CRMDAYOD.newTable  ExtrapMethod=Clip  InternalRulePriority=Speed  RndMeth=Simplest  InputSameDT=on
  Constant : Constant
  Sum : Sum  Inputs=-+|
  eoeff : Outport
  eieff : Outport  Port=2
  wires:
  Sum/1 -> eieff/1
  CRMDAYOD_M/1 -> eoeff/1, Sum/1
  Constant/1 -> Sum/2
  Bus Selector/1 -> CRMDAYOD_M/1  "<mach_nd>"
  AeroIn_Bus/1 -> Bus Selector/1

== system ADMIRE/Aircraft/Aerodynamics/RollMomentCoefficient/MachRegion3/Crmbasic ==
  Constant : Constant  Value=0
  Crmbasic : Outport
  wires:
  Constant/1 -> Crmbasic/1

== system ADMIRE/Aircraft/Aerodynamics/RollMomentCoefficient/MachRegion3/Crmbde ==
  in_bus : Inport
  Bus Selector : BusSelector  OutputSignals=AeroIn_Bus.angleOfAttack_deg,AeroIn_Bus.dN,AeroIn_Bus.dEI,AeroIn_Bus.angleOfSideslip_deg,AeroIn_Bus.dEY,eieff,eoeff,AeroIn_Bus.mach_nd
  Crmbde_ : Subsystem
  Crmbde : Outport
  wires:
  Bus Selector/8 -> Crmbde_/8(mach_nd)  "<mach_nd>"
  Bus Selector/7 -> Crmbde_/7(eoeff)  "<eoeff>"
  Bus Selector/6 -> Crmbde_/6(eieff)  "<eieff>"
  Bus Selector/5 -> Crmbde_/5(dEY)  "<dEY>"
  Bus Selector/4 -> Crmbde_/4(angleOfSideslip_deg)  "<angleOfSideslip_deg>"
  Bus Selector/3 -> Crmbde_/3(dEI)  "<dEI>"
  Bus Selector/2 -> Crmbde_/2(dN)  "<dN>"
  Bus Selector/1 -> Crmbde_/1(angleOfAttack_deg)  "<angleOfAttack_deg>"
  Crmbde_/1(Crmbde) -> Crmbde/1
  in_bus/1 -> Bus Selector/1  "in_bus"

== system ADMIRE/Aircraft/Aerodynamics/RollMomentCoefficient/MachRegion3/Crmbdle ==
  in_bus : Inport
  Bus Selector : BusSelector  OutputSignals=AeroIn_Bus.angleOfAttack_deg,AeroIn_Bus.dEI,AeroIn_Bus.mach_nd,AeroIn_Bus.dEY,eieff,eoeff,AeroIn_Bus.angleOfSideslip_deg,AeroIn_Bus.lef_deg
  Crmbdle_ : Subsystem
  Crmbdle : Outport
  wires:
  Bus Selector/1 -> Crmbdle_/1(angleOfAttack_deg)  "<angleOfAttack_deg>"
  Bus Selector/2 -> Crmbdle_/2(dEI)  "<dEI>"
  Bus Selector/3 -> Crmbdle_/3(mach_nd)  "<mach_nd>"
  Bus Selector/4 -> Crmbdle_/4(dEY)  "<dEY>"
  Bus Selector/5 -> Crmbdle_/5(eieff)  "<eieff>"
  Bus Selector/6 -> Crmbdle_/6(eoeff)  "<eoeff>"
  Bus Selector/7 -> Crmbdle_/7(angleOfSideslip_deg)  "<angleOfSideslip_deg>"
  Bus Selector/8 -> Crmbdle_/8(dLE)  "<lef_deg>"
  Crmbdle_/1(Crmbdle) -> Crmbdle/1
  in_bus/1 -> Bus Selector/1  "in_bus"

== system ADMIRE/Aircraft/Aerodynamics/RollMomentCoefficient/MachRegion3/Crmbdn ==
  in_bus : Inport
  Bus Selector : BusSelector  OutputSignals=AeroIn_Bus.dN,AeroIn_Bus.mach_nd,AeroIn_Bus.angleOfSideslip_deg
  Crmbdn_ : Subsystem
  Crmbdn : Outport
  wires:
  Bus Selector/3 -> Crmbdn_/3(angleOfSideslip_deg)  "<angleOfSideslip_deg>"
  Bus Selector/1 -> Crmbdn_/1(dN)  "<dN>"
  Bus Selector/2 -> Crmbdn_/2(mach_nd)  "<mach_nd>"
  in_bus/1 -> Bus Selector/1  "in_bus"
  Crmbdn_/1(Crmbdn) -> Crmbdn/1

== system ADMIRE/Aircraft/Aerodynamics/RollMomentCoefficient/MachRegion3/Crmbeta ==
  in_bus : Inport
  Bus Selector : BusSelector  OutputSignals=AeroIn_Bus.mach_nd,AeroIn_Bus.angleOfAttack_deg,AeroIn_Bus.angleOfSideslip_deg,AeroIn_Bus.qacorr
  Crmbeta_ : Subsystem
  Crmbeta : Outport
  wires:
  Bus Selector/2 -> Crmbeta_/2(angleOfAttack_deg)  "<angleOfAttack_deg>"
  Bus Selector/1 -> Crmbeta_/1(mach_nd)  "<mach_nd>"
  Bus Selector/3 -> Crmbeta_/3(angleOfSideslip_deg)  "<angleOfSideslip_deg>"
  Bus Selector/4 -> Crmbeta_/4(qacorr)  "<qacorr>"
  in_bus/1 -> Bus Selector/1  "in_bus"
  Crmbeta_/1(Crmbeta) -> Crmbeta/1

== system ADMIRE/Aircraft/Aerodynamics/RollMomentCoefficient/MachRegion3/Crmbetad ==
  in_bus : Inport
  Bus Selector : BusSelector  OutputSignals=AeroIn_Bus.angleOfAttack_deg,AeroIn_Bus.mach_nd,AeroIn_Bus.betad
  Crmbetad_ : Subsystem
  Crmbetad : Outport
  wires:
  Bus Selector/3 -> Crmbetad_/3(betad)  "<betad>"
  Bus Selector/1 -> Crmbetad_/1(angleOfAttack_deg)  "<angleOfAttack_deg>"
  Bus Selector/2 -> Crmbetad_/2(mach_nd)  "<mach_nd>"
  in_bus/1 -> Bus Selector/1  "in_bus"
  Crmbetad_/1(Crmbetad) -> Crmbetad/1

== system ADMIRE/Aircraft/Aerodynamics/RollMomentCoefficient/MachRegion3/Crmblg ==
  in_bus : Inport
  Bus Selector : BusSelector  OutputSignals=AeroIn_Bus.lg_bool,AeroIn_Bus.angleOfAttack_deg,AeroIn_Bus.angleOfSideslip_deg
  Crmblg_ : Subsystem
  Crmblg : Outport
  wires:
  Bus Selector/3 -> Crmblg_/3(angleOfSideslip_deg)  "<angleOfSideslip_deg>"
  Bus Selector/2 -> Crmblg_/2(angleOfAttack_deg)  "<angleOfAttack_deg>"
  Bus Selector/1 -> Crmblg_/1(dLG)  "<lg_bool>"
  in_bus/1 -> Bus Selector/1  "in_bus"
  Crmblg_/1(Crmblg) -> Crmblg/1

== system ADMIRE/Aircraft/Aerodynamics/RollMomentCoefficient/MachRegion3/Crmdai ==
  in_bus : Inport
  Bus Selector : BusSelector  OutputSignals=AeroIn_Bus.angleOfAttack_deg,AeroIn_Bus.dAI,AeroIn_Bus.mach_nd,AeroIn_Bus.dEI,eieff,AeroIn_Bus.qacorr
  Crmdai_ : Subsystem
  Crmdai : Outport
  wires:
  Bus Selector/6 -> Crmdai_/6(qacorr)  "<qacorr>"
  Bus Selector/5 -> Crmdai_/5(eieff)  "<eieff>"
  Bus Selector/4 -> Crmdai_/4(dEI)  "<dEI>"
  Bus Selector/3 -> Crmdai_/3(mach_nd)  "<mach_nd>"
  Bus Selector/2 -> Crmdai_/2(dAI)  "<dAI>"
  Bus Selector/1 -> Crmdai_/1(angleOfAttack_deg)  "<angleOfAttack_deg>"
  in_bus/1 -> Bus Selector/1  "in_bus"
  Crmdai_/1(Crmdai) -> Crmdai/1

== system ADMIRE/Aircraft/Aerodynamics/RollMomentCoefficient/MachRegion3/Crmdaib ==
  Constant : Constant  Value=0
  Crmdaib : Outport
  wires:
  Constant/1 -> Crmdaib/1

== system ADMIRE/Aircraft/Aerodynamics/RollMomentCoefficient/MachRegion3/Crmday ==
  in_bus : Inport
  Bus Selector : BusSelector  OutputSignals=AeroIn_Bus.angleOfAttack_deg,AeroIn_Bus.dAY,AeroIn_Bus.mach_nd,AeroIn_Bus.dEY,eoeff,AeroIn_Bus.qacorr
  Crmday_ : Subsystem
  Crmday : Outport
  wires:
  Bus Selector/1 -> Crmday_/1(angleOfAttack_deg)  "<angleOfAttack_deg>"
  Bus Selector/2 -> Crmday_/2(dAI)  "<dAY>"
  Bus Selector/3 -> Crmday_/3(mach_nd)  "<mach_nd>"
  Bus Selector/4 -> Crmday_/4(dEI)  "<dEY>"
  Bus Selector/5 -> Crmday_/5(eieff)  "<eoeff>"
  Bus Selector/6 -> Crmday_/6(qacorr)  "<qacorr>"
  Crmday_/1(Crmdai) -> Crmday/1
  in_bus/1 -> Bus Selector/1  "in_bus"

== system ADMIRE/Aircraft/Aerodynamics/RollMomentCoefficient/MachRegion3/Crmdayb ==
  Constant : Constant  Value=0
  Crmdayb : Outport
  wires:
  Constant/1 -> Crmdayb/1

== system ADMIRE/Aircraft/Aerodynamics/RollMomentCoefficient/MachRegion3/Crmdna ==
  in_bus : Inport
  Bus Selector : BusSelector  OutputSignals=AeroIn_Bus.angleOfAttack_deg,AeroIn_Bus.dNA
  Crmdna_ : Subsystem
  Crmdna : Outport
  wires:
  Bus Selector/2 -> Crmdna_/2(dNA)  "<dNA>"
  Bus Selector/1 -> Crmdna_/1(angleOfAttack_deg)  "<angleOfAttack_deg>"
  Crmdna_/1(Crmdna) -> Crmdna/1
  in_bus/1 -> Bus Selector/1  "in_bus"

== system ADMIRE/Aircraft/Aerodynamics/RollMomentCoefficient/MachRegion3/Crmdr ==
  in_bus : Inport
  Bus Selector : BusSelector  OutputSignals=AeroIn_Bus.qacorr,AeroIn_Bus.mach_nd,AeroIn_Bus.rud_deg
  Crmdr_ : Subsystem
  Crmdr : Outport
  wires:
  Bus Selector/3 -> Crmdr_/3(dR)  "<rud_deg>"
  Bus Selector/2 -> Crmdr_/2(mach_nd)  "<mach_nd>"
  Bus Selector/1 -> Crmdr_/1(qacorr)  "<qacorr>"
  Crmdr_/1(Crmdr) -> Crmdr/1
  in_bus/1 -> Bus Selector/1  "in_bus"

== system ADMIRE/Aircraft/Aerodynamics/RollMomentCoefficient/MachRegion3/Crmp ==
  in_bus : Inport
  Bus Selector : BusSelector  OutputSignals=AeroIn_Bus.angleOfAttack_deg,AeroIn_Bus.mach_nd,AeroIn_Bus.pc,AeroIn_Bus.qacorr
  Crmp_ : Subsystem
  Crmp : Outport
  wires:
  Bus Selector/4 -> Crmp_/4(qacorr)  "<qacorr>"
  Bus Selector/3 -> Crmp_/3(pc)  "<pc>"
  Bus Selector/2 -> Crmp_/2(mach_nd)  "<mach_nd>"
  Bus Selector/1 -> Crmp_/1(angleOfAttack_deg)  "<angleOfAttack_deg>"
  Crmp_/1(Crmp) -> Crmp/1
  in_bus/1 -> Bus Selector/1  "in_bus"

== system ADMIRE/Aircraft/Aerodynamics/RollMomentCoefficient/MachRegion3/Crmpbeta ==
  Crmpbeta_ : Constant  Value=0
  Crmpbeta : Outport
  wires:
  Crmpbeta_/1 -> Crmpbeta/1

== system ADMIRE/Aircraft/Aerodynamics/RollMomentCoefficient/MachRegion3/Crmr ==
  in_bus : Inport
  Bus Selector : BusSelector  OutputSignals=AeroIn_Bus.angleOfAttack_deg,AeroIn_Bus.mach_nd,AeroIn_Bus.rc
  Crmr_ : Subsystem
  Crmr : Outport
  wires:
  Bus Selector/3 -> Crmr_/3(rc)  "<rc>"
  Bus Selector/2 -> Crmr_/2(mach_nd)  "<mach_nd>"
  Bus Selector/1 -> Crmr_/1(angleOfAttack_deg)  "<angleOfAttack_deg>"
  Crmr_/1(Crmr) -> Crmr/1
  in_bus/1 -> Bus Selector/1  "in_bus"

== system ADMIRE/Aircraft/Aerodynamics/RollMomentCoefficient/MachRegion3/Crmrbeta ==
  Crmrbeta_ : Constant  Value=0
  Crmrbeta : Outport
  wires:
  Crmrbeta_/1 -> Crmrbeta/1

== system ADMIRE/Aircraft/Aerodynamics/RollMomentCoefficient/MachRegion3/Crmrde ==
  in_bus : Inport
  Bus Selector : BusSelector  OutputSignals=AeroIn_Bus.mach_nd,AeroIn_Bus.angleOfAttack_deg,AeroIn_Bus.rc,AeroIn_Bus.dEI,eieff,AeroIn_Bus.dEY,eoeff
  Crmrde_ : Subsystem
  Crmrde : Outport
  wires:
  Bus Selector/1 -> Crmrde_/1(mach_nd)  "<mach_nd>"
  Bus Selector/2 -> Crmrde_/2(angleOfAttack_deg)  "<angleOfAttack_deg>"
  Bus Selector/3 -> Crmrde_/3(rc)  "<rc>"
  Bus Selector/4 -> Crmrde_/4(dEI)  "<dEI>"
  Bus Selector/5 -> Crmrde_/5(eieff)  "<eieff>"
  Bus Selector/6 -> Crmrde_/6(dEY)  "<dEY>"
  Bus Selector/7 -> Crmrde_/7(eoeff)  "<eoeff>"
  Crmrde_/1(Crmrde) -> Crmrde/1
  in_bus/1 -> Bus Selector/1  "in_bus"

== system ADMIRE/Aircraft/Aerodynamics/RollMomentCoefficient/MachRegion3/eoeff1 ==
  AeroIn_Bus : Inport
  Bus Selector : BusSelector  OutputSignals=mach_nd
  CRMDAYOD_M : Lookup_n-D  NumberOfTableDimensions=1  BreakpointsForDimension1=admireDB.aerodata_asym_ext.CRMDAYOD.breakpoints.M  BreakpointsForDimension3=[5, 7]  Table=admireDB.aerodata_asym_ext.CRMDAYOD.newTable  ExtrapMethod=Clip  InternalRulePriority=Speed  RndMeth=Simplest  InputSameDT=on
  Constant : Constant
  Sum : Sum  Inputs=-+|
  eoeff : Outport
  eieff : Outport  Port=2
  wires:
  Sum/1 -> eieff/1
  CRMDAYOD_M/1 -> eoeff/1, Sum/1
  Constant/1 -> Sum/2
  Bus Selector/1 -> CRMDAYOD_M/1  "<mach_nd>"
  AeroIn_Bus/1 -> Bus Selector/1

== system ADMIRE/Aircraft/Aerodynamics/RollMomentCoefficient/MachRegion4/Crmbasic ==
  Constant : Constant  Value=0
  Crmbasic : Outport
  wires:
  Constant/1 -> Crmbasic/1
